simulink model "s0433"  (Simulink 7.0)
settings: Solver=ode45  SolverMode=SingleTasking  StartTime=0.0  StopTime=10  FixedStep=1  MaxStep=1  RelTol=1e-3  AbsTol=1e-6
values from neighbouring files (symbols this model uses):
  Gsnen = Gs.den{1}    [m0404Bsp.m]
  Gszae = Gs.num{1}    [m0404Bsp.m]
  Kpr = 10    [m0108d.m]    (also in m0109b.m = 1; m0113c.m; m0404Bsp.m = 3)
  Tt = .4    (= 0.4)    [m0108d.m]    (also in m0259.m = 1; m0314.m = 2.13; m0322.m = 0.8; m0326.m = 4)
  w_steptime = w_steptime-t0A    (= 6)    [m0404Bsp.m]
  wdach_ = wdach    (= 1)    [m0404Bsp.m]
  z_steptime = z_steptime-t0A    (= 1)    [m0404Bsp.m]
  zdach_ = zdach    (= 1)    [m0404Bsp.m]
undefined symbols (not defined in the file or in its folder): Tr, xD
libraries: simulink x1
settings Model: Creator=froriep  LastModifiedBy=froriep
settings DataIOCC: LimitDataPoints=off  SaveOutput=off  SaveTime=off
settings OptimizationCC: BooleanDataType=off
settings DebuggingCC: SaveWithParameterizedLinksMsg=none  SignalResolutionControl=TryResolveAllWithWarning  SolverPrmCheckMsg=none  MultiTaskDSMMsg=warning  MultiTaskCondExecSysMsg=none  StrictBusMsg=None
settings HardwareCC: TargetUnknown=on
settings RTWCC: IncludeERTFirstTime=on

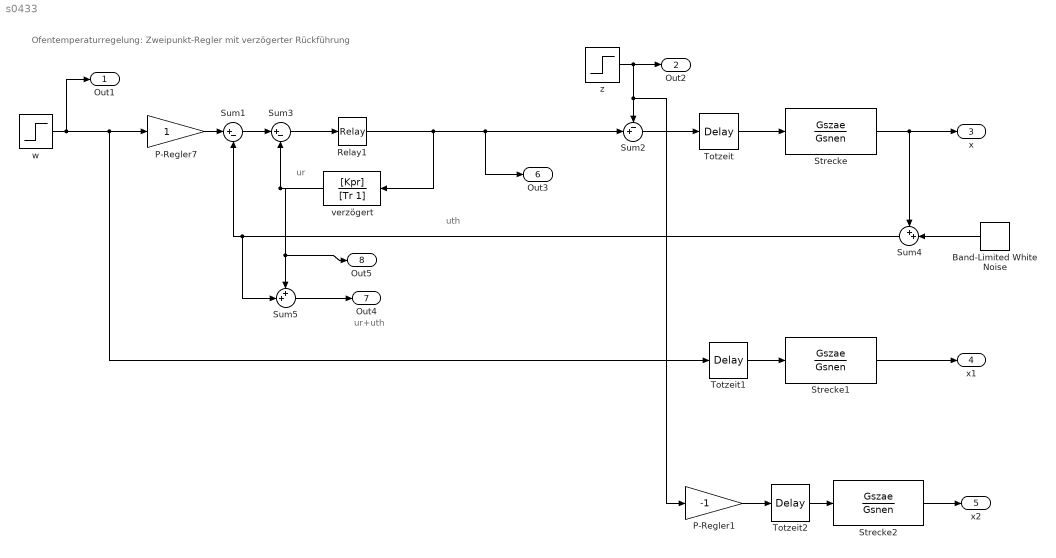
== system s0433 ==
  note: Ofentemperaturregelung: Zweipunkt-Regler mit verzögerter Rückführung
  note: ur+uth
  note: ur
  note: uth
  Band-Limited White Noise : simulink/Sources/Band-Limited White Noise  Orientation=left  SystemSampleTime=-1  Cov=Rauschen  Ts=.01  seed=[23341]
  P-Regler1 : Gain  Gain=-1  ParameterDataType=sfix(16)  ParameterScaling=2^0  OutDataType=sfix(16)  OutScaling=2^0
  P-Regler7 : Gain  ParameterDataType=sfix(16)  ParameterScaling=2^0  OutDataType=sfix(16)  OutScaling=2^0
  Relay1 : Relay  OnSwitchValue=xD/2  OffSwitchValue=-xD/2  OnOutputValue=Yh  OutDataType=sfix(16)  OutScaling=2^0
  Strecke : TransferFcn  Numerator=Gszae  Denominator=Gsnen
  Strecke1 : TransferFcn  Numerator=Gszae  Denominator=Gsnen
  Strecke2 : TransferFcn  Numerator=Gszae  Denominator=Gsnen
  Sum1 : Sum  Inputs=|+-  SaturateOnIntegerOverflow=on  InputSameDT=on
  Sum2 : Sum  Inputs=-+|  SaturateOnIntegerOverflow=on  InputSameDT=on
  Sum3 : Sum  Inputs=|+-  SaturateOnIntegerOverflow=on  InputSameDT=on
  Sum4 : Sum  Orientation=left  Inputs=++|  SaturateOnIntegerOverflow=on  InputSameDT=on
  Sum5 : Sum  Inputs=++|  SaturateOnIntegerOverflow=on  InputSameDT=on
  Totzeit : TransportDelay  DelayTime=Tt
  Totzeit1 : TransportDelay  DelayTime=Tt
  Totzeit2 : TransportDelay  DelayTime=Tt
  verzögert : TransferFcn  Orientation=left  Numerator=[Kpr]  Denominator=[Tr 1]
  w : Step  Time=w_steptime  After=wdach_  SampleTime=0
  z : Step  Time=z_steptime  After=zdach_  SampleTime=0
  Out1 : Outport  OutDataType=sfix(16)  OutScaling=2^0
  Out2 : Outport  Port=2  OutDataType=sfix(16)  OutScaling=2^0
  x : Outport  Port=3  OutDataType=sfix(16)  OutScaling=2^0
  x1 : Outport  Port=4  OutDataType=sfix(16)  OutScaling=2^0
  x2 : Outport  Port=5  OutDataType=sfix(16)  OutScaling=2^0
  Out3 : Outport  Port=6  OutDataType=sfix(16)  OutScaling=2^0
  Out4 : Outport  Port=7  OutDataType=sfix(16)  OutScaling=2^0
  Out5 : Outport  Port=8  OutDataType=sfix(16)  OutScaling=2^0
  wires:
  z/1 -> Out2/1, Sum2/1, P-Regler1/1
  w/1 -> Out1/1, P-Regler7/1, Totzeit1/1
  Strecke/1 -> x/1, Sum4/1
  Sum4/1 -> Sum1/2, Sum5/2
  Band-Limited White Noise/1 -> Sum4/2
  Sum1/1 -> Sum3/1
  Totzeit/1 -> Strecke/1
  Sum2/1 -> Totzeit/1
  Sum3/1 -> Relay1/1
  verzögert/1 -> Sum3/2, Sum5/1, Out5/1
  Relay1/1 -> verzögert/1, Sum2/2, Out3/1
  P-Regler7/1 -> Sum1/1
  Strecke1/1 -> x1/1
  Totzeit1/1 -> Strecke1/1
  Strecke2/1 -> x2/1
  Totzeit2/1 -> Strecke2/1
  P-Regler1/1 -> Totzeit2/1
  Sum5/1 -> Out4/1
